simulink model "downlink_8c4t"  (Simulink 8.7)
settings: Solver=VariableStepDiscrete  StartTime=0.0  StopTime=20000  RelTol=1e-3
PreLoadFcn:
  | % Run the setup script when the model is opened
  | setup_downlink_8c4t;
InitFcn:
  | % Run the setup script again just before the
  | % model is run, so that any updates made
  | % after opening are applied.
  | 
  | setup_downlink_8c4t;
  | 
  | 
  | %% DSPBuilder Start
  | alt_dspbuilder_update_model(bdroot)
  | %% DSPBuilder End
values from neighbouring files (symbols this model uses):
  LUTS =     [downlink_8c4t_luts2.mat]
undefined symbols (not defined in the file or in its folder): DUC_LINEUP_param, value
libraries: DSPBAModelBus x44, DSPBABase x9, pipereg_lib x6, blind_cfr_lib x4, hduc_lib x4, dpd_lib x4, simulink x2, mixer_lib x2, lduc_lib x2, summer_4c4t_lib x2, DSPBAPrim x1
(part 2 of 2)

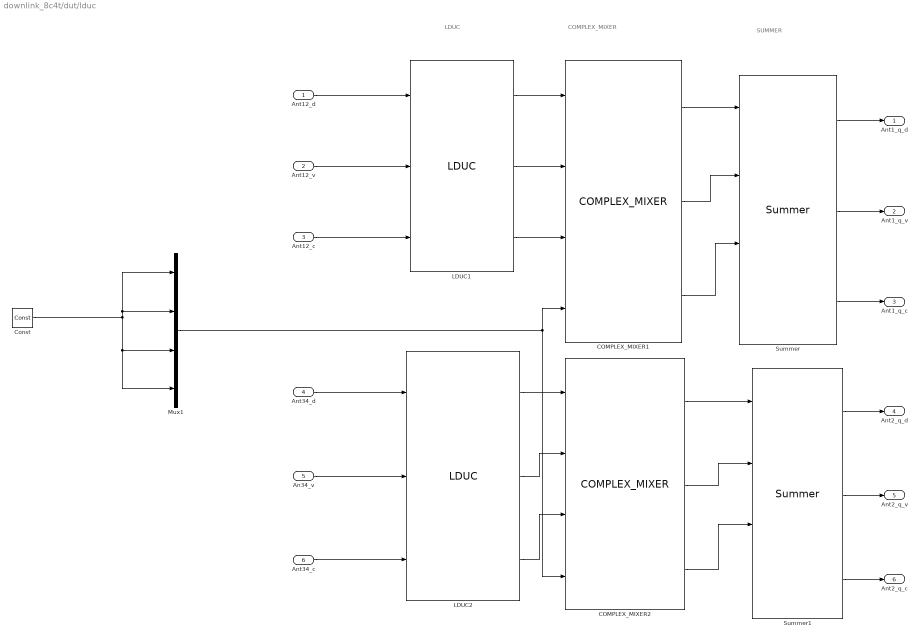
== system downlink_8c4t/dut/lduc ==
  note: LDUC
  note: COMPLEX_MIXER
  note: SUMMER
  Ant12_d : Inport
  Ant12_v : Inport  Port=2
  Ant12_c : Inport  Port=3
  Ant34_d : Inport  Port=4
  An34_v : Inport  Port=5
  Ant34_c : Inport  Port=6
  COMPLEX_MIXER1 : mixer_lib/COMPLEX_MIXER  CM_clock_margin=DUC_LINEUP_param.ClockMargin  CM_NCO_sample_rate=DUC_LINEUP_param.NCO.SampleRate  CM_NCO_accumulator_bit_width=DUC_LINEUP_param.NCO.Acumulater_bit_wid  CM_NCO_frequency_word=DUC_LINEUP_param.NCO_ant12.Freq_word  CM_NCO_base_addr=DUC_LINEUP_param.NCO_ant12.base_addr  CM_NCO_data_type=DUC_LINEUP_param.NCO.Data_type  CM_NCO_scaling_value=DUC_LINEUP_param.NCO.scaling_value  CM_sample_rate=DUC_LINEUP_param.CM.SampleRate  CM_complex_channels=DUC_LINEUP_param.CM.No_Of_Complex_chan  CM_complex_freq=DUC_LINEUP_param.CM.No_Of_Complex_Freq  CM_output_word_length=DUC_LINEUP_param.output_word_length  CM_output_fraction_length=DUC_LINEUP_param.output_fraction_length  CM_scale_multiplication_factor=DUC_CM_multiplication_factor  CM_scale_left_shift_factor=DUC_CM_Number_of_bits_to_shift_left  CM_NCO_phase=DUC_CM_NCO_phase  CM_NCO_sync=DUC_CM_NCO_sync
      link override ComplexMixer: latency=4
      link override ComplexMixer_Scale: latency=0
      link override Complex_NCO: expSFDR=96.32  accumPrecision=+/- 3.6621  phaseIncrInMHz="[-30  -10   10   30  -30  -10   10   30  -30  -10   10   30  -30  -10   10   30]"  outWidth=4  tableSize=8  latency=19
      link override Delay Module/ChannelOut: value=2  packetBeginEnabled=off  latency=1
      link override NCO Delay Matching/ChannelOut: latency=0
      link override NCO_Delay_Matching /ChannelOut: latency=2
      link override PipeReg_2in1/ChannelOut: value=2  packetBeginEnabled=off  latency=2
      link override PipeReg_2in5/ChannelOut: value=2  packetBeginEnabled=off  latency=2
  COMPLEX_MIXER2 : mixer_lib/COMPLEX_MIXER  CM_clock_margin=DUC_LINEUP_param.ClockMargin  CM_NCO_sample_rate=DUC_LINEUP_param.NCO.SampleRate  CM_NCO_accumulator_bit_width=DUC_LINEUP_param.NCO.Acumulater_bit_wid  CM_NCO_frequency_word=DUC_LINEUP_param.NCO_ant34.Freq_word  CM_NCO_base_addr=DUC_LINEUP_param.NCO_ant34.base_addr  CM_NCO_data_type=DUC_LINEUP_param.NCO.Data_type  CM_NCO_scaling_value=DUC_LINEUP_param.NCO.scaling_value  CM_sample_rate=DUC_LINEUP_param.CM.SampleRate  CM_complex_channels=DUC_LINEUP_param.CM.No_Of_Complex_chan  CM_complex_freq=DUC_LINEUP_param.CM.No_Of_Complex_Freq  CM_output_word_length=DUC_LINEUP_param.output_word_length  CM_output_fraction_length=DUC_LINEUP_param.output_fraction_length  CM_scale_multiplication_factor=DUC_CM_multiplication_factor  CM_scale_left_shift_factor=DUC_CM_Number_of_bits_to_shift_left  CM_NCO_phase=DUC_CM_NCO_phase  CM_NCO_sync=DUC_CM_NCO_sync
      link override ComplexMixer: latency=4
      link override ComplexMixer_Scale: latency=0
      link override Complex_NCO: expSFDR=96.32  accumPrecision=+/- 3.6621  phaseIncrInMHz="[-30  -10   10   30  -30  -10   10   30  -30  -10   10   30  -30  -10   10   30]"  outWidth=4  tableSize=8  latency=19
      link override Delay Module/ChannelOut: value=2  packetBeginEnabled=off  latency=1
      link override NCO Delay Matching/ChannelOut: latency=0
      link override NCO_Delay_Matching /ChannelOut: latency=2
      link override PipeReg_2in1/ChannelOut: value=2  packetBeginEnabled=off  latency=2
      link override PipeReg_2in5/ChannelOut: value=2  packetBeginEnabled=off  latency=2
  Const : DSPBAPrim/Const  primtype=const  nInputs=0  nOutputs=1  omode=boolean  otype=sfix(16)  scale=2^-15  rndmethod=Unbiased  factor=1  satmethod=Symmetric  shift_vec=[0 1 2 -1]  value=0  inPortNames=['+'; '+';]  outPortNames=[' ']  dspbaimage=dspba_prim.jpg  text=fprintf('%s', num2str(value));  style=Optimised  visibilities=8 + 1024  floatPrecision=float32_m23  version=20120820
  LDUC1 : lduc_lib/LDUC  Clock_Margin=DUC_LINEUP_param.ClockMargin  chan_filter_SampleRate=DUC_LINEUP_param.chan_filter.SampleRate  chan_filter_ChanCount=DUC_LINEUP_param.chan_filter.ChanCount  chan_filter_coeffs=DUC_LINEUP_param.chan_filter.coeffs(1,:)  chan_filter_base_addr=DUC_LINEUP_param.chan_filter.base_addr1  HB_filt4_SampleRate=DUC_LINEUP_param.HB_filt4.SampleRate  HB_filt_Interpolation=DUC_LINEUP_param.HB_filt4.Interpolation  HB_filt4_ChanCount=DUC_LINEUP_param.HB_filt4.ChanCount  HB_filt4_coeffs=DUC_LINEUP_param.HB_filt4.coeffs(1,:)  HB_filt4_base_addr=DUC_LINEUP_param.HB_filt4.base_addr1  HB_filt5_SampleRate=DUC_LINEUP_param.HB_filt5.SampleRate  HB_filt5_Interpolation=DUC_LINEUP_param.HB_filt5.Interpolation  HB_filt5_ChanCount=DUC_LINEUP_param.HB_filt5.ChanCount  HB_filt5_coeffs=DUC_LINEUP_param.HB_filt5.coeffs(1,:)  HB_filt5_base_addr=DUC_LINEUP_param.HB_filt5.base_addr1  Pipe_Reg=2  CH_Multiplication_fact=1  CH_Bits_to_Left_shift=0  HB4_Multiplication_fact=1  HB4_Bits_to_left_shift=1  HB5_Multiplication_fact=1  HB5_Bits_to_Left_shift=1  output_word_length=DUC_LINEUP_param.output_word_length  output_fraction_length=DUC_LINEUP_param.output_fraction_length
      link override Channel_Filter/ChannelIm: latency=4
      link override Channel_Filter/ChannelRe: latency=4
      link override Channel_Filter/scale_ChannelIm: latency=3
      link override Channel_Filter/scale_ChannelRe: latency=3
      link override HB4/HB4Im: latency=15
      link override HB4/HB4Re: latency=15
      link override HB4/scale_HB4Im: latency=3
      link override HB4/scale_HB4Re: latency=3
      link override HB5/HB5Im: latency=11
      link override HB5/HB5Re: latency=11
      link override HB5/scale_HB5Im: latency=3
      link override HB5/scale_HB5Re: latency=3
  LDUC2 : lduc_lib/LDUC  Clock_Margin=DUC_LINEUP_param.ClockMargin  chan_filter_SampleRate=DUC_LINEUP_param.chan_filter.SampleRate  chan_filter_ChanCount=DUC_LINEUP_param.chan_filter.ChanCount  chan_filter_coeffs=DUC_LINEUP_param.chan_filter.coeffs(1,:)  chan_filter_base_addr=DUC_LINEUP_param.chan_filter.base_addr2  HB_filt4_SampleRate=DUC_LINEUP_param.HB_filt4.SampleRate  HB_filt_Interpolation=DUC_LINEUP_param.HB_filt4.Interpolation  HB_filt4_ChanCount=DUC_LINEUP_param.HB_filt4.ChanCount  HB_filt4_coeffs=DUC_LINEUP_param.HB_filt4.coeffs(1,:)  HB_filt4_base_addr=DUC_LINEUP_param.HB_filt4.base_addr2  HB_filt5_SampleRate=DUC_LINEUP_param.HB_filt5.SampleRate  HB_filt5_Interpolation=DUC_LINEUP_param.HB_filt5.Interpolation  HB_filt5_ChanCount=DUC_LINEUP_param.HB_filt5.ChanCount  HB_filt5_coeffs=DUC_LINEUP_param.HB_filt5.coeffs(1,:)  HB_filt5_base_addr=DUC_LINEUP_param.HB_filt5.base_addr2  Pipe_Reg=2  CH_Multiplication_fact=1  CH_Bits_to_Left_shift=0  HB4_Multiplication_fact=1  HB4_Bits_to_left_shift=1  HB5_Multiplication_fact=1  HB5_Bits_to_Left_shift=1  output_word_length=DUC_LINEUP_param.output_word_length  output_fraction_length=DUC_LINEUP_param.output_fraction_length
      link override Channal_Filter/SingleRateFIR: latency=4
      link override Channal_Filter/scale_SingleRateFIR: latency=4
      link override Channel_Filter/ChannelIm: latency=4
      link override Channel_Filter/ChannelRe: latency=4
      link override Channel_Filter/scale_ChannelIm: latency=3
      link override Channel_Filter/scale_ChannelRe: latency=3
      link override HB4/HB4Im: latency=15
      link override HB4/HB4Re: latency=15
      link override HB4/HB_filter4: latency=14
      link override HB4/scale_HB4Im: latency=3
      link override HB4/scale_HB4Re: latency=3
      link override HB4/scale_HB_filter4: latency=4
      link override HB5/HB5Im: latency=11
      link override HB5/HB5Re: latency=11
      link override HB5/HB_filter5: latency=10
      link override HB5/scale_HB5Im: latency=3
      link override HB5/scale_HB5Re: latency=3
      link override HB5/scale_HB_filter5: latency=4
      link override PipeReg1/ChannelOut: value=1  packetBeginEnabled=off  latency=2
      link override PipeReg2/ChannelOut: value=1  packetBeginEnabled=off  latency=2
      link override PipeReg3/ChannelOut: value=1  packetBeginEnabled=off  latency=2
      link override PipeReg4/ChannelOut: value=1  packetBeginEnabled=off  latency=2
      link override PipeReg5/ChannelOut: value=1  packetBeginEnabled=off  latency=2
      link override PipeReg6/ChannelOut: value=1  packetBeginEnabled=off  latency=2
      link override PipeReg7/ChannelOut: value=1  packetBeginEnabled=off  latency=2
      link override PipeReg8/ChannelOut: value=1  packetBeginEnabled=off  latency=2
  Mux1 : Mux
  Summer : summer_4c4t_lib/Summer  ClockMargin=DUC_LINEUP_param.ClockMargin  output_word_length=DUC_LINEUP_param.output_word_length  output_fraction_length=DUC_LINEUP_param.output_fraction_length  Summer_Multiplication_fact=DUC_SUMMER_multiplication_factor  Summer_left_shift_fact=DUC_SUMMER_Number_of_bits_to_shift_left  Pipeline_stages=2  Latency=40
      link override Antenna_Summer/ChannelOut: latency=3
      link override scale_Antenna_Summer: latency=6
  Summer1 : summer_4c4t_lib/Summer  ClockMargin=DUC_LINEUP_param.ClockMargin  output_word_length=DUC_LINEUP_param.output_word_length  output_fraction_length=DUC_LINEUP_param.output_fraction_length  Summer_Multiplication_fact=DUC_SUMMER_multiplication_factor  Summer_left_shift_fact=DUC_SUMMER_Number_of_bits_to_shift_left  Pipeline_stages=2  Latency=40
      link override Antenna_Summer/ChannelOut: latency=3
      link override scale_Antenna_Summer: latency=6
  Ant1_q_d : Outport
  Ant1_q_v : Outport  Port=2
  Ant1_q_c : Outport  Port=3
  Ant2_q_d : Outport  Port=4
  Ant2_q_v : Outport  Port=5
  Ant2_q_c : Outport  Port=6
  wires:
  Ant12_v/1 -> LDUC1/2
  Ant34_c/1 -> LDUC2/3
  Ant34_d/1 -> LDUC2/1
  Ant12_c/1 -> LDUC1/3
  Summer1/1 -> Ant2_q_d/1
  Summer/2 -> Ant1_q_v/1
  Summer/1 -> Ant1_q_d/1
  Summer/3 -> Ant1_q_c/1
  An34_v/1 -> LDUC2/2
  Summer1/3 -> Ant2_q_c/1
  Ant12_d/1 -> LDUC1/1
  Summer1/2 -> Ant2_q_v/1
  LDUC1/1 -> COMPLEX_MIXER1/1
  LDUC1/2 -> COMPLEX_MIXER1/2
  LDUC1/3 -> COMPLEX_MIXER1/3
  COMPLEX_MIXER1/3 -> Summer/3
  COMPLEX_MIXER1/2 -> Summer/2
  COMPLEX_MIXER1/1 -> Summer/1
  LDUC2/1 -> COMPLEX_MIXER2/1
  LDUC2/2 -> COMPLEX_MIXER2/2
  LDUC2/3 -> COMPLEX_MIXER2/3
  COMPLEX_MIXER2/2 -> Summer1/2
  COMPLEX_MIXER2/1 -> Summer1/1
  COMPLEX_MIXER2/3 -> Summer1/3
  Mux1/1 -> COMPLEX_MIXER2/4, COMPLEX_MIXER1/4
  Const/1 -> Mux1/3, Mux1/4, Mux1/1, Mux1/2

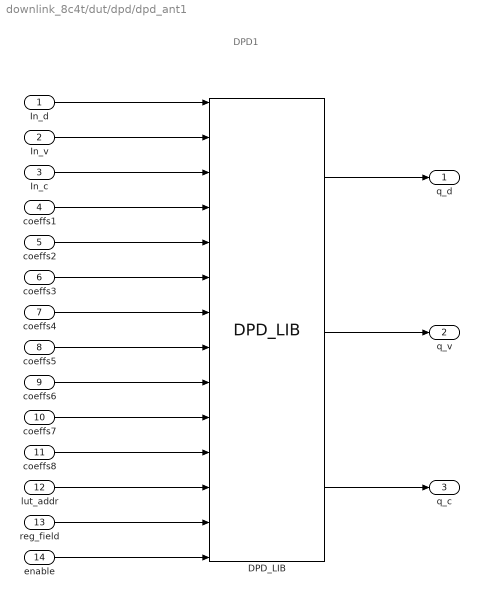
== system downlink_8c4t/dut/dpd/dpd_ant1 ==
  note: DPD1
  In_d : Inport
  In_v : Inport  Port=2
  In_c : Inport  Port=3
  coeffs1 : Inport  Port=4
  coeffs2 : Inport  Port=5
  coeffs3 : Inport  Port=6
  coeffs4 : Inport  Port=7
  coeffs5 : Inport  Port=8
  coeffs6 : Inport  Port=9
  coeffs7 : Inport  Port=10
  coeffs8 : Inport  Port=11
  lut_addr : Inport  Port=12
  reg_field : Inport  Port=13
  enable : Inport  Port=14
  DPD_LIB : dpd_lib/DPD_LIB  CoefWidth=16  Coeff_fractionwidth=11  DataWidth=16  fractionwidth=15  Lateny=60  ClockMargin=DUC_LINEUP_param.ClockMargin_DPD  Pipeline_stages=2  LutContent=LUTS.ENTRIES
      link override dpd/ChannelOut1: latency=61
  q_d : Outport
  q_v : Outport  Port=2
  q_c : Outport  Port=3
  wires:
  coeffs1/1 -> DPD_LIB/4
  In_c/1 -> DPD_LIB/3
  coeffs2/1 -> DPD_LIB/5
  coeffs8/1 -> DPD_LIB/11
  In_v/1 -> DPD_LIB/2
  In_d/1 -> DPD_LIB/1
  lut_addr/1 -> DPD_LIB/12
  coeffs6/1 -> DPD_LIB/9
  coeffs5/1 -> DPD_LIB/8
  coeffs4/1 -> DPD_LIB/7
  coeffs3/1 -> DPD_LIB/6
  enable/1 -> DPD_LIB/14
  coeffs7/1 -> DPD_LIB/10
  DPD_LIB/1 -> q_d/1
  DPD_LIB/3 -> q_c/1
  reg_field/1 -> DPD_LIB/13
  DPD_LIB/2 -> q_v/1

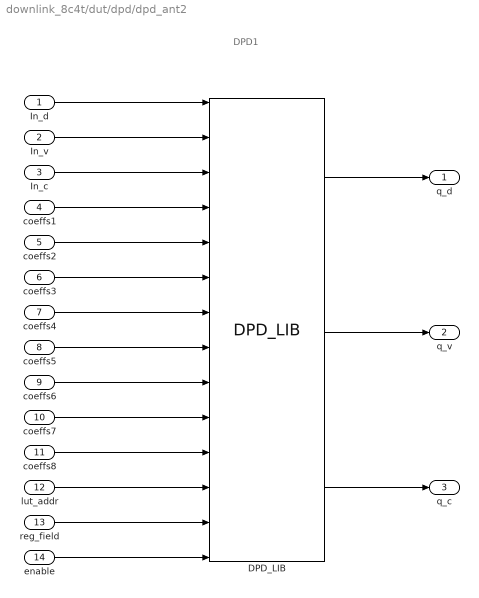
== system downlink_8c4t/dut/dpd/dpd_ant2 ==
  note: DPD1
  In_d : Inport
  In_v : Inport  Port=2
  In_c : Inport  Port=3
  coeffs1 : Inport  Port=4
  coeffs2 : Inport  Port=5
  coeffs3 : Inport  Port=6
  coeffs4 : Inport  Port=7
  coeffs5 : Inport  Port=8
  coeffs6 : Inport  Port=9
  coeffs7 : Inport  Port=10
  coeffs8 : Inport  Port=11
  lut_addr : Inport  Port=12
  reg_field : Inport  Port=13
  enable : Inport  Port=14
  DPD_LIB : dpd_lib/DPD_LIB  CoefWidth=16  Coeff_fractionwidth=11  DataWidth=16  fractionwidth=15  Lateny=60  ClockMargin=DUC_LINEUP_param.ClockMargin_DPD  Pipeline_stages=2  LutContent=LUTS.ENTRIES
      link override dpd/ChannelOut1: latency=61
  q_d : Outport
  q_v : Outport  Port=2
  q_c : Outport  Port=3
  wires:
  coeffs1/1 -> DPD_LIB/4
  In_c/1 -> DPD_LIB/3
  coeffs2/1 -> DPD_LIB/5
  coeffs8/1 -> DPD_LIB/11
  In_v/1 -> DPD_LIB/2
  In_d/1 -> DPD_LIB/1
  lut_addr/1 -> DPD_LIB/12
  coeffs6/1 -> DPD_LIB/9
  coeffs5/1 -> DPD_LIB/8
  coeffs4/1 -> DPD_LIB/7
  coeffs3/1 -> DPD_LIB/6
  enable/1 -> DPD_LIB/14
  coeffs7/1 -> DPD_LIB/10
  DPD_LIB/1 -> q_d/1
  DPD_LIB/3 -> q_c/1
  reg_field/1 -> DPD_LIB/13
  DPD_LIB/2 -> q_v/1

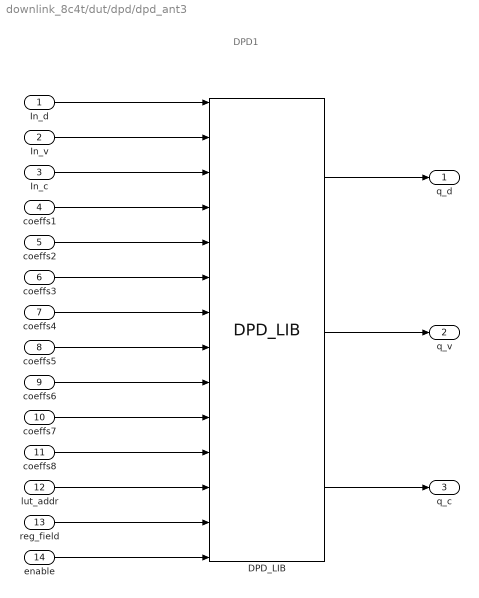
== system downlink_8c4t/dut/dpd/dpd_ant3 ==
  note: DPD1
  In_d : Inport
  In_v : Inport  Port=2
  In_c : Inport  Port=3
  coeffs1 : Inport  Port=4
  coeffs2 : Inport  Port=5
  coeffs3 : Inport  Port=6
  coeffs4 : Inport  Port=7
  coeffs5 : Inport  Port=8
  coeffs6 : Inport  Port=9
  coeffs7 : Inport  Port=10
  coeffs8 : Inport  Port=11
  lut_addr : Inport  Port=12
  reg_field : Inport  Port=13
  enable : Inport  Port=14
  DPD_LIB : dpd_lib/DPD_LIB  CoefWidth=16  Coeff_fractionwidth=11  DataWidth=16  fractionwidth=15  Lateny=60  ClockMargin=DUC_LINEUP_param.ClockMargin_DPD  Pipeline_stages=2  LutContent=LUTS.ENTRIES
      link override dpd/ChannelOut1: latency=61
  q_d : Outport
  q_v : Outport  Port=2
  q_c : Outport  Port=3
  wires:
  coeffs1/1 -> DPD_LIB/4
  In_c/1 -> DPD_LIB/3
  coeffs2/1 -> DPD_LIB/5
  coeffs8/1 -> DPD_LIB/11
  In_v/1 -> DPD_LIB/2
  In_d/1 -> DPD_LIB/1
  lut_addr/1 -> DPD_LIB/12
  coeffs6/1 -> DPD_LIB/9
  coeffs5/1 -> DPD_LIB/8
  coeffs4/1 -> DPD_LIB/7
  coeffs3/1 -> DPD_LIB/6
  enable/1 -> DPD_LIB/14
  coeffs7/1 -> DPD_LIB/10
  DPD_LIB/1 -> q_d/1
  DPD_LIB/3 -> q_c/1
  reg_field/1 -> DPD_LIB/13
  DPD_LIB/2 -> q_v/1

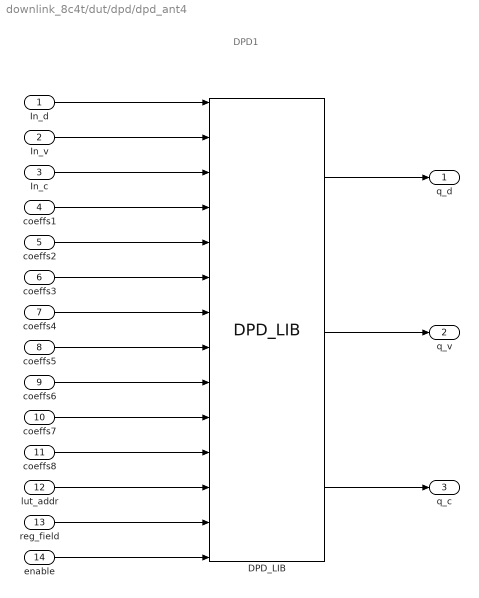
== system downlink_8c4t/dut/dpd/dpd_ant4 ==
  note: DPD1
  In_d : Inport
  In_v : Inport  Port=2
  In_c : Inport  Port=3
  coeffs1 : Inport  Port=4
  coeffs2 : Inport  Port=5
  coeffs3 : Inport  Port=6
  coeffs4 : Inport  Port=7
  coeffs5 : Inport  Port=8
  coeffs6 : Inport  Port=9
  coeffs7 : Inport  Port=10
  coeffs8 : Inport  Port=11
  lut_addr : Inport  Port=12
  reg_field : Inport  Port=13
  enable : Inport  Port=14
  DPD_LIB : dpd_lib/DPD_LIB  CoefWidth=16  Coeff_fractionwidth=11  DataWidth=16  fractionwidth=15  Lateny=60  ClockMargin=DUC_LINEUP_param.ClockMargin_DPD  Pipeline_stages=2  LutContent=LUTS.ENTRIES
      link override dpd/ChannelOut1: latency=61
  q_d : Outport
  q_v : Outport  Port=2
  q_c : Outport  Port=3
  wires:
  coeffs1/1 -> DPD_LIB/4
  In_c/1 -> DPD_LIB/3
  coeffs2/1 -> DPD_LIB/5
  coeffs8/1 -> DPD_LIB/11
  In_v/1 -> DPD_LIB/2
  In_d/1 -> DPD_LIB/1
  lut_addr/1 -> DPD_LIB/12
  coeffs6/1 -> DPD_LIB/9
  coeffs5/1 -> DPD_LIB/8
  coeffs4/1 -> DPD_LIB/7
  coeffs3/1 -> DPD_LIB/6
  enable/1 -> DPD_LIB/14
  coeffs7/1 -> DPD_LIB/10
  DPD_LIB/1 -> q_d/1
  DPD_LIB/3 -> q_c/1
  reg_field/1 -> DPD_LIB/13
  DPD_LIB/2 -> q_v/1
